simulink model "dampedSpring"  (Simulink 4.00)
settings: Solver=ode45  StartTime=0.0  StopTime=0.2  RelTol=1e-3
settings Model: LastModifiedBy=JimmyL  SingleTaskRateTransMsg=warning  CheckForMatrixSingularity=warning  UnnecessaryDatatypeConvMsg=warning  SignalLabelMismatchMsg=warning  VectorMatrixConversionMsg=warning  SfunCompatibilityCheckMsg=warning

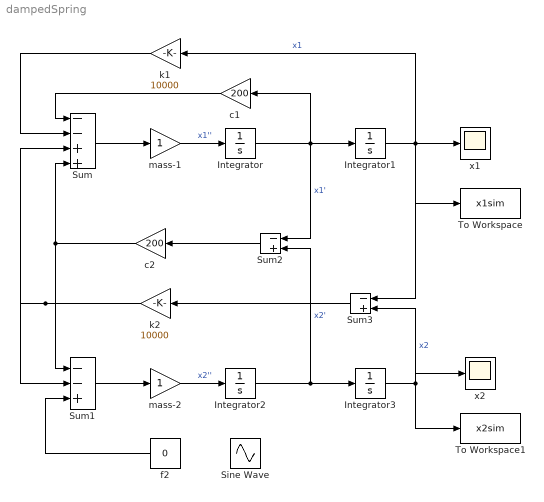
== system dampedSpring ==
  Integrator : Integrator  ExternalReset=none  InitialConditionSource=internal  InitialCondition=0  LimitOutput=off  UpperSaturationLimit=inf  LowerSaturationLimit=-inf  ShowSaturationPort=off  ShowStatePort=off  AbsoluteTolerance=auto
  Integrator1 : Integrator  ExternalReset=none  InitialConditionSource=internal  InitialCondition=0  LimitOutput=off  UpperSaturationLimit=inf  LowerSaturationLimit=-inf  ShowSaturationPort=off  ShowStatePort=off  AbsoluteTolerance=auto
  Integrator2 : Integrator  ExternalReset=none  InitialConditionSource=internal  InitialCondition=0  LimitOutput=off  UpperSaturationLimit=inf  LowerSaturationLimit=-inf  ShowSaturationPort=off  ShowStatePort=off  AbsoluteTolerance=auto
  Integrator3 : Integrator  ExternalReset=none  InitialConditionSource=internal  InitialCondition=0.01  LimitOutput=off  UpperSaturationLimit=inf  LowerSaturationLimit=-inf  ShowSaturationPort=off  ShowStatePort=off  AbsoluteTolerance=auto
  Sine Wave : Sin  SineType=Time-based  Amplitude=0.1  Bias=0  Frequency=10  Phase=0  Samples=10  SampleTime=0  Offset=0
  Sum : Sum  Inputs=--++  SaturateOnIntegerOverflow=on
  Sum1 : Sum  Inputs=--+  SaturateOnIntegerOverflow=on
  Sum2 : Sum  Orientation=left  Inputs=-+  SaturateOnIntegerOverflow=on
  Sum3 : Sum  Orientation=left  Inputs=-+  SaturateOnIntegerOverflow=on
  To Workspace : ToWorkspace  VariableName=x1sim  SampleTime=1e-3  SaveFormat=Array
  To Workspace1 : ToWorkspace  VariableName=x2sim  SampleTime=1e-3  SaveFormat=Array
  c1 : Gain  Orientation=left  Gain=200  Multiplication=Element-wise(K.*u)  SaturateOnIntegerOverflow=on
  c2 : Gain  Description=c2  Orientation=left  Gain=200  Multiplication=Element-wise(K.*u)  SaturateOnIntegerOverflow=on
  f2 : Constant  Orientation=left  Value=0
  k1 : Gain  Orientation=left  Gain=10000  Multiplication=Element-wise(K.*u)  SaturateOnIntegerOverflow=on
  k2 : Gain  Orientation=left  Gain=10000  Multiplication=Element-wise(K.*u)  SaturateOnIntegerOverflow=on
  mass-1 : Gain  Gain=1  Multiplication=Element-wise(K.*u)  SaturateOnIntegerOverflow=on
  mass-2 : Gain  Gain=1  Multiplication=Element-wise(K.*u)  SaturateOnIntegerOverflow=on
  x1 : Scope
      settings: TimeRange=0.2  YMin=-0.001  YMax=0.0015  SaveToWorkspace=off  SaveName=ScopeData  LimitDataPoints=on  MaxDataPoints=5000  SampleTime=1e-4
  x2 : Scope
      settings: TimeRange=0.2  YMin=-0.002  YMax=0.01  SaveToWorkspace=off  LimitDataPoints=on  MaxDataPoints=5000  SampleTime=1e-4
  wires:
  Sum/1 -> mass-1/1
  mass-1/1 -> Integrator/1  "x1''"
  c2/1 -> Sum/4, Sum1/1
  Integrator/1 -> Integrator1/1, Sum2/1, c1/1  "x1'"
  k1/1 -> Sum/2
  Integrator1/1 -> k1/1, Sum3/1, x1/1, To Workspace/1  "x1"
  Sum1/1 -> mass-2/1
  mass-2/1 -> Integrator2/1  "x2''"
  Integrator2/1 -> Integrator3/1, Sum2/2  "x2'"
  Integrator3/1 -> Sum3/2, x2/1, To Workspace1/1  "x2"
  Sum2/1 -> c2/1
  Sum3/1 -> k2/1
  k2/1 -> Sum1/2, Sum/3
  c1/1 -> Sum/1
  f2/1 -> Sum1/3
